simulink model "Car"  (R2025b)
settings: Solver=VariableStepAuto  StartTime=0.0  StopTime=10.0  RelTol=1e-3
undefined symbols (not defined in the file): b, M
settings Model: Creator=vvpai9  LastModifiedBy=vvpai9

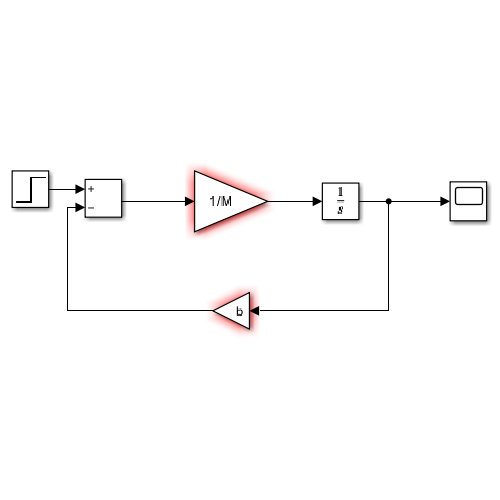
[thumbnail: Simulink's stored preview of the top-level diagram]
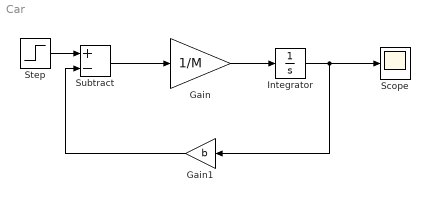
== system Car ==
  Gain : Gain  Gain=1/M
  Gain1 : Gain  Gain=b
  Integrator : Integrator
  Scope : Scope
  Step : Step  SampleTime=0
  Subtract : Sum  Inputs=+-
  wires:
  Step/1 -> Subtract/1
  Subtract/1 -> Gain/1
  Gain/1 -> Integrator/1
  Integrator/1 -> Gain1/1, Scope/1
  Gain1/1 -> Subtract/2
